simulink model "Part3"  (R2018a)
settings: Solver=VariableStepAuto  StartTime=0.0  StopTime=1000  RelTol=1e-3
values from neighbouring files (symbols this model uses):
  A = [-0.322, 0.052, 0.028, -1.12, 0.002 ... (first row only)    [InitialisePart1.m]
  B = [0; 0; 0; 0; -7.5]    [InitialisePart1.m]
  C = [ 0   0  1   0 ... (first row only)    [InitialisePart1.m]
  d = 1.5*deg2rad    (= 0.0261799387799)    [InitialisePart1.m]    (also in init.m)
  g = 9.81    [InitialisePart1.m]    (also in init.m = -9.81)
  k_d_phi = (2*zeta*omega_n-a_phi_1)/a_phi_2    [InitialisePart1.m]    (also in init.m)
  k_i_khi = (V_g/g)*(omega_x)^2    [InitialisePart1.m]    (also in init.m)
  k_i_phi = -1    [InitialisePart1.m]    (also in init.m = 1)
  k_p_khi = (V_g/g)*2*zeta_x*omega_x    [InitialisePart1.m]    (also in init.m)
  k_p_phi = delta_a_max/e_max*sign(a_phi_2)    [InitialisePart1.m]    (also in init.m)
  roll_v = (0.2*deg2rad)^2    (= 1.21846967915e-05)    [InitialisePart1.m]
  V_g = V_a    (= 161.111111111)    [InitialisePart1.m]    (also in init.m)
  yaw_v = (0.2*deg2rad)^2    (= 1.21846967915e-05)    [InitialisePart1.m]
settings Model: Creator=martimos  LastModifiedBy=martin
settings CodeAppCC: StateflowObjectComments=on

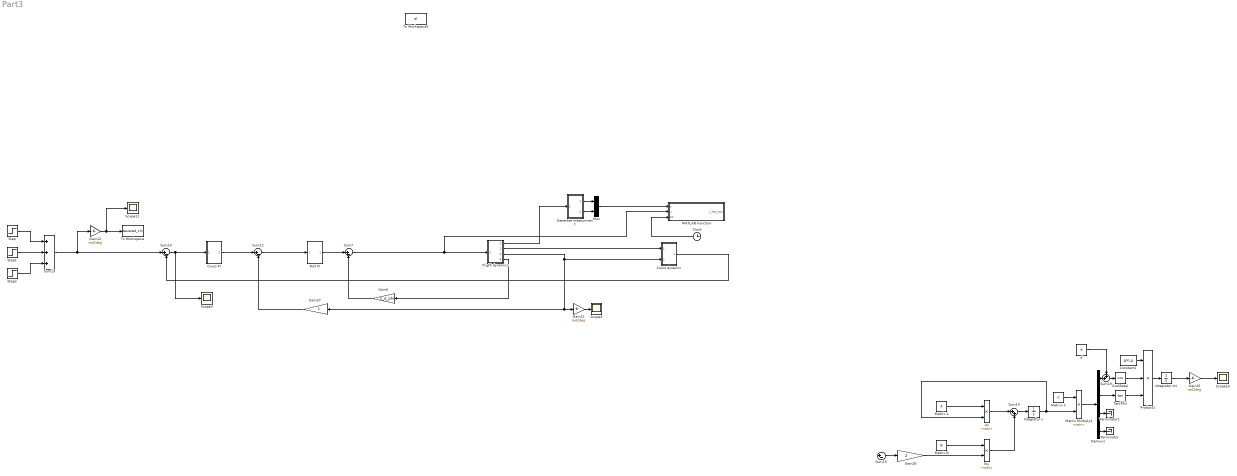
== system Part3 ==
  Ax : Product  Multiplication=Matrix(*)
  Bu : Product  Multiplication=Matrix(*)
  Clock : Clock
  Constant1 : Constant  Value=g/V_g
  Cos(Beta) : Trigonometry  Operator=cos
  Cours PI : Subsystem
  Cours dynamic : Subsystem
  Demux1 : Demux
  Flight dynamics : Subsystem
  Gain12 : Gain  Gain=rad2deg
  Gain22 : Gain  Gain=rad2deg
  Gain25 : Gain  Gain=rad2deg
  Gain26 : Gain  Gain=2
  Gain27 : Gain
  Gain6 : Gain  Gain=k_d_phi
  Generate measurment : Subsystem
  "Integrator chi " : Integrator
  "Integrator x " : Integrator
  MATLAB Function : MATLAB Function  TreatAsAtomicUnit=on
  Matriix C : Constant  Value=C
  Matrix A : Constant  Value=A
  Matrix B : Constant  Value=B
  Matrix Multiply4 : Product  Multiplication=Matrix(*)
  Mux : Mux  Inputs=2
  Product1 : Product  Inputs=3
  Roll PI : Subsystem
  Scope{3..4,10..11} (4 alike) : Scope
  Step : Step  Time=5  After=2*deg2rad  SampleTime=0
  Step1 : Step  Time=50  After=-2*deg2rad  SampleTime=0
  Step2 : Step  Time=150  After=-4*deg2rad  SampleTime=0
  Sum{7,10,12,15} (4 alike) : Sum  Inputs=|+-
  Sum13 : Sum  Inputs=+++
  Sum14 : Sum  Inputs=|++
  Sum19 : Sum  Inputs=++|
  Tan(Phi) : Trigonometry  Operator=tan
  Terminator : Terminator
  Terminator1 : Terminator
  To Workspace : ToWorkspace  VariableName=desiered_chi  SaveFormat=Timeseries  SampleTime=-1
  To Workspace5 : ToWorkspace  VariableName=al  SaveFormat=Timeseries  SampleTime=-1
  d : Constant  Value=d
  wires:
  Gain6/1 -> Sum7/2
  Sum10/1 -> Scope3/1, Cours PI/1(In1)
  Sum13/1 -> Gain12/1, Sum10/1
  Step/1 -> Sum13/1
  Step1/1 -> Sum13/2
  Step2/1 -> Sum13/3
  Gain12/1 -> To Workspace/1, Scope11/1
  Gain22/1 -> Scope4/1
  Matrix A/1 -> Ax/1
  Matrix B/1 -> Bu/1
  Ax/1 -> Sum14/1
  Bu/1 -> Sum14/2
  Sum14/1 -> "Integrator x "/1
  "Integrator x "/1 -> Ax/2, Matrix Multiply4/2
  Matriix C/1 -> Matrix Multiply4/1
  Gain25/1 -> Scope10/1
  Matrix Multiply4/1 -> Demux1/1
  Demux1/4 -> Terminator/1
  Constant1/1 -> Product1/1
  Demux1/2 -> Tan(Phi)/1
  Cos(Beta)/1 -> Product1/2
  Tan(Phi)/1 -> Product1/3
  Product1/1 -> "Integrator chi "/1
  "Integrator chi "/1 -> Gain25/1
  Sum19/1 -> Cos(Beta)/1
  d/1 -> Sum19/1
  Sum15/1 -> Gain26/1
  Demux1/3 -> Terminator1/1
  Gain26/1 -> Bu/2
  Demux1/1 -> Sum19/2
  Gain27/1 -> Sum12/2
  Cours PI/1(Out1) -> Sum12/1
  Sum12/1 -> Roll PI/1(In1)
  Roll PI/1(Out1) -> Sum7/1
  Cours dynamic/1(Out1) -> Sum10/2
  Flight dynamics/3(Out3) -> Cours dynamic/2(In2), Gain22/1, Gain27/1
  Sum7/1 -> MATLAB Function/2(u), Flight dynamics/1(In1)
  Flight dynamics/2(Out2) -> Cours dynamic/1(In1)
  Flight dynamics/4(Out4) -> Gain6/1
  Flight dynamics/1(Out1) -> Generate measurment/1(In1)
  Generate measurment/1(Out3) -> Mux/1
  Generate measurment/2(Out4) -> Mux/2
  Mux/1 -> MATLAB Function/1(y)
  Clock/1 -> MATLAB Function/3(tid)

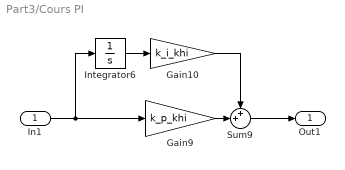
== system Part3/Cours PI ==
  In1 : Inport
  Gain10 : Gain  Gain=k_i_khi
  Gain9 : Gain  Gain=k_p_khi
  Integrator6 : Integrator
  Sum9 : Sum  Inputs=++|
  Out1 : Outport
  wires:
  Gain9/1 -> Sum9/2
  In1/1 -> Integrator6/1, Gain9/1
  Sum9/1 -> Out1/1
  Gain10/1 -> Sum9/1
  Integrator6/1 -> Gain10/1

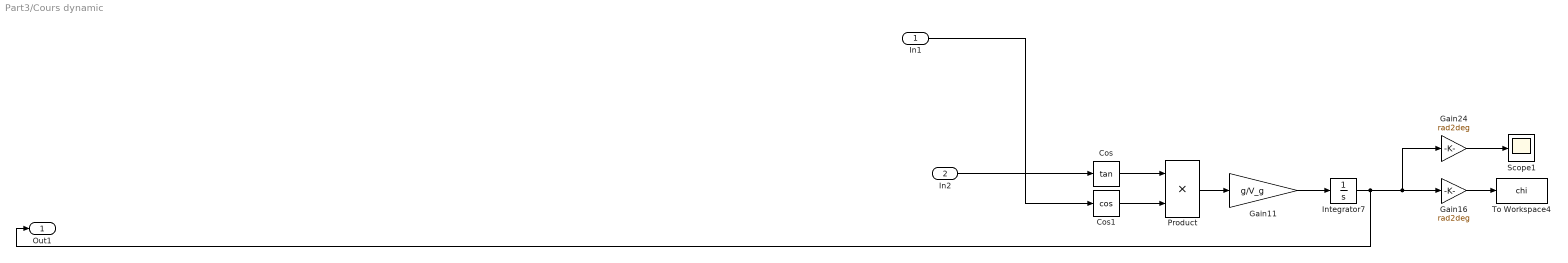
== system Part3/Cours dynamic ==
  In1 : Inport
  In2 : Inport  Port=2
  Cos : Trigonometry  Operator=tan
  Cos1 : Trigonometry  Operator=cos
  Gain11 : Gain  Gain=g/V_g
  Gain16 : Gain  Gain=rad2deg
  Gain24 : Gain  Gain=rad2deg
  Integrator7 : Integrator
  Product : Product
  Scope1 : Scope
  To Workspace4 : ToWorkspace  VariableName=chi  SaveFormat=Timeseries  SampleTime=-1
  Out1 : Outport
  wires:
  Cos/1 -> Product/1
  Gain16/1 -> To Workspace4/1
  Cos1/1 -> Product/2
  In1/1 -> Cos1/1
  Gain11/1 -> Integrator7/1
  Integrator7/1 -> Out1/1, Gain16/1, Gain24/1
  Product/1 -> Gain11/1
  Gain24/1 -> Scope1/1
  In2/1 -> Cos/1

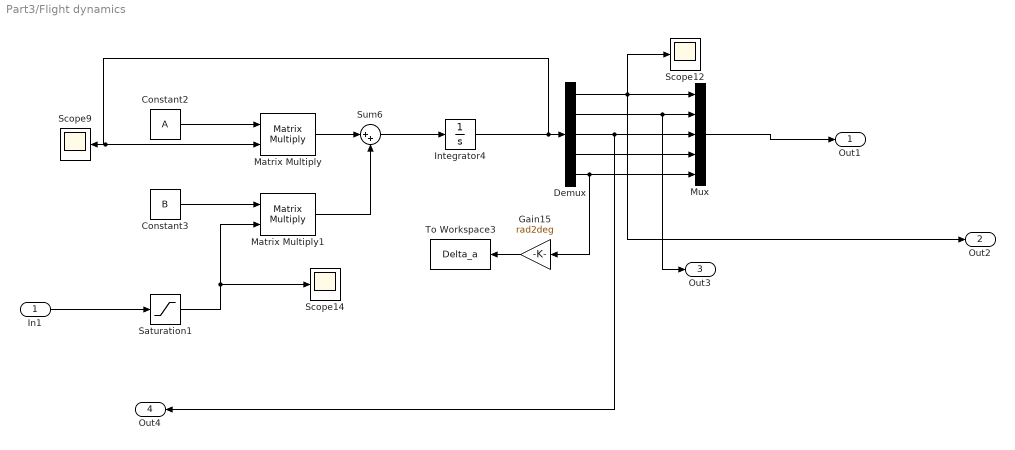
== system Part3/Flight dynamics ==
  In1 : Inport
  Constant2 : Constant  Value=A
  Constant3 : Constant  Value=B
  Demux : Demux  Outputs=5
  Gain15 : Gain  Gain=rad2deg
  Integrator4 : Integrator
  Matrix Multiply : Product  Multiplication=Matrix(*)
  Matrix Multiply1 : Product  Multiplication=Matrix(*)
  Mux : Mux  Inputs=5
  Saturation1 : Saturate  UpperLimit=0.523333  LowerLimit=-0.52333
  Scope12 : Scope
  Scope14 : Scope
  Scope9 : Scope
  Sum6 : Sum  Inputs=|++
  To Workspace3 : ToWorkspace  VariableName=Delta_a  SaveFormat=Timeseries  SampleTime=-1
  Out1 : Outport
  Out2 : Outport  Port=2
  Out3 : Outport  Port=3
  Out4 : Outport  Port=4
  wires:
  Matrix Multiply/1 -> Sum6/1
  Demux/4 -> Mux/4
  Sum6/1 -> Integrator4/1
  Integrator4/1 -> Demux/1, Scope9/1, Matrix Multiply/2
  Demux/3 -> Out4/1, Mux/3
  Demux/1 -> Out2/1, Mux/1, Scope12/1
  Saturation1/1 -> Scope14/1, Matrix Multiply1/2
  Matrix Multiply1/1 -> Sum6/2
  Mux/1 -> Out1/1
  Demux/2 -> Out3/1, Mux/2
  Demux/5 -> Gain15/1, Mux/5
  Gain15/1 -> To Workspace3/1
  In1/1 -> Saturation1/1
  Constant2/1 -> Matrix Multiply/1
  Constant3/1 -> Matrix Multiply1/1

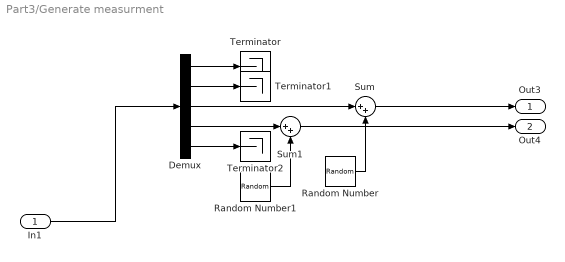
== system Part3/Generate measurment ==
  In1 : Inport
  Demux : Demux  Outputs=5
  Random Number : RandomNumber  Variance=roll_v  SampleTime=0.1
  Random Number1 : RandomNumber  Variance=yaw_v  SampleTime=0.1
  Sum : Sum  Inputs=|++
  Sum1 : Sum  Inputs=|++
  Terminator : Terminator
  Terminator1 : Terminator
  Terminator2 : Terminator
  Out3 : Outport
  Out4 : Outport  Port=2
  wires:
  Random Number1/1 -> Sum1/2
  Demux/3 -> Sum/1
  Demux/2 -> Terminator1/1
  Random Number/1 -> Sum/2
  Demux/4 -> Sum1/1
  Demux/5 -> Terminator2/1
  In1/1 -> Demux/1
  Sum1/1 -> Out4/1
  Sum/1 -> Out3/1
  Demux/1 -> Terminator/1

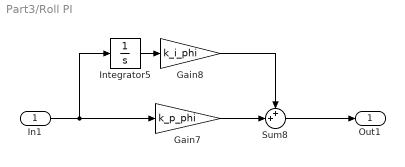
== system Part3/Roll PI ==
  In1 : Inport
  Gain7 : Gain  Gain=k_p_phi
  Gain8 : Gain  Gain=k_i_phi
  Integrator5 : Integrator
  Sum8 : Sum  Inputs=++|
  Out1 : Outport
  wires:
  Integrator5/1 -> Gain8/1
  In1/1 -> Integrator5/1, Gain7/1
  Sum8/1 -> Out1/1
  Gain7/1 -> Sum8/2
  Gain8/1 -> Sum8/1

== matlab function Part3/MATLAB Function ==
  data: y input; u input; x_hat_new output; tid input
function x_hat_new = fcn(y,u, tid)

K = P_0*C'*(C*P_0C'+R)^(-1);
x_hat = x_0+K(y-C*x_0);
P_hat = (eye(4) -K*C)*P_0*(eye(4)-K*C)' + K*R*K';

x_0 = PHI*x_hat+DELTA*u;
P_0 = PHI*P_hat*PHI'+GAMA*Q*GAMA';

x_hat_new = x_hat;
